simulink model "regulator_model"  (R2021b)
settings: Solver=VariableStepAuto  StartTime=0.0  StopTime=0.25  RelTol=1e-3
values from neighbouring files (symbols this model uses):
  Bm = 8.8e-5    (= 8.8e-05)    [regulator_parameters.m]
  Jm = 8.5e-5    (= 8.5e-05)    [regulator_parameters.m]
  Ke = 0.022    [regulator_parameters.m]
  La = 0.00027    [regulator_parameters.m]
  Ra = 0.12    [regulator_parameters.m]
  TL = 0    [regulator_parameters.m]
  Va = 12    [regulator_parameters.m]
libraries: simulink_extras x2
settings Model: Creator=sacka  LastModifiedBy=sacka

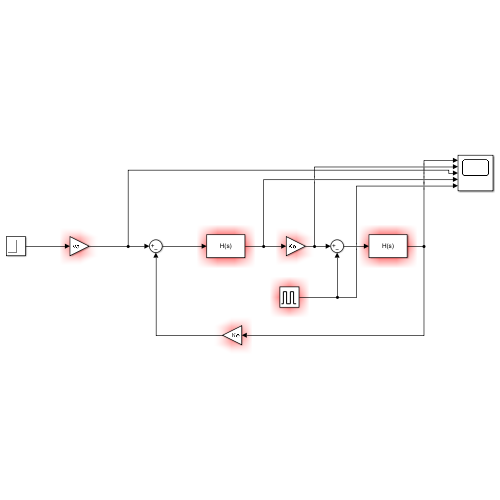
[thumbnail: Simulink's stored preview of the top-level diagram]
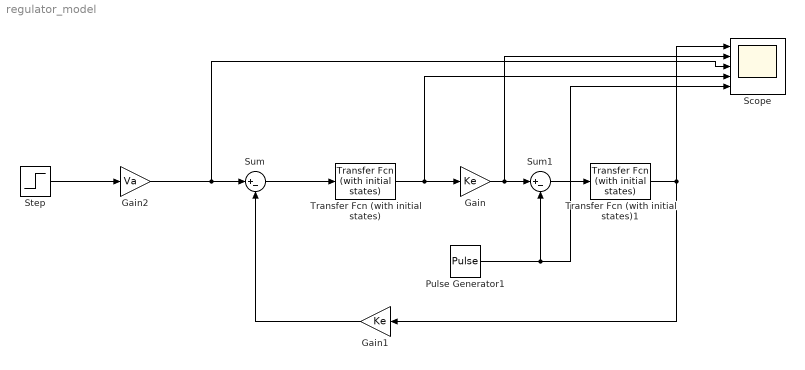
== system regulator_model ==
  Gain : Gain  Gain=Ke
  Gain1 : Gain  Gain=Ke
  Gain2 : Gain  Gain=Va
  Pulse Generator1 : DiscretePulseGenerator  PulseType=Time based  Amplitude=TL  Period=30  PulseWidth=90  PhaseDelay=6
  Scope : Scope  NumInputPorts=5
  Step : Step  Before=1  SampleTime=0
  Sum : Sum  Inputs=|+-
  Sum1 : Sum  Inputs=|+-
  Transfer Fcn (with initial states) : simulink_extras/Additional Linear/Transfer Fcn (with initial states)  N=[1]  D=[La Ra]  X0=0
  Transfer Fcn (with initial states)1 : simulink_extras/Additional Linear/Transfer Fcn (with initial states)  N=[1]  D="[Jm  Bm]"  X0=0
  wires:
  Sum/1 -> Transfer Fcn (with initial states)/1
  Transfer Fcn (with initial states)/1 -> Scope/4, Gain/1
  Pulse Generator1/1 -> Scope/5, Sum1/2
  Gain/1 -> Scope/2, Sum1/1
  Gain1/1 -> Sum/2
  Sum1/1 -> Transfer Fcn (with initial states)1/1
  Transfer Fcn (with initial states)1/1 -> Scope/1, Gain1/1
  Gain2/1 -> Scope/3, Sum/1
  Step/1 -> Gain2/1
